simulink library "arducopter_library"  (R2015a)
settings: Solver=ode45  StartTime=0.0  StopTime=10.0  RelTol=1e-3
values from neighbouring files (symbols this model uses):
  dt = 0.01    [arducopter_initialization.m]    (also in startup.m)
  use_ff = true    [arducopter_initialization.m]    (also in startup.m)
undefined symbols (not defined in the file or in its folder): P
libraries: simulink x3, arducopter_library x2
settings Model: CovSaveCumulativeToWorkspaceVar=on  Creator=anne  LastModifiedBy=pa872d
settings DataIOCC: SaveFormat=Dataset
settings HardwareCC: ProdBitPerPointer=64  ProdLargestAtomicFloat=Float  ProdIntDivRoundTo=Zero  ProdEndianess=LittleEndian  ProdHWDeviceType=Specified
settings ModelReferenceCC: PropagateSignalLabelsOutOfModel=on

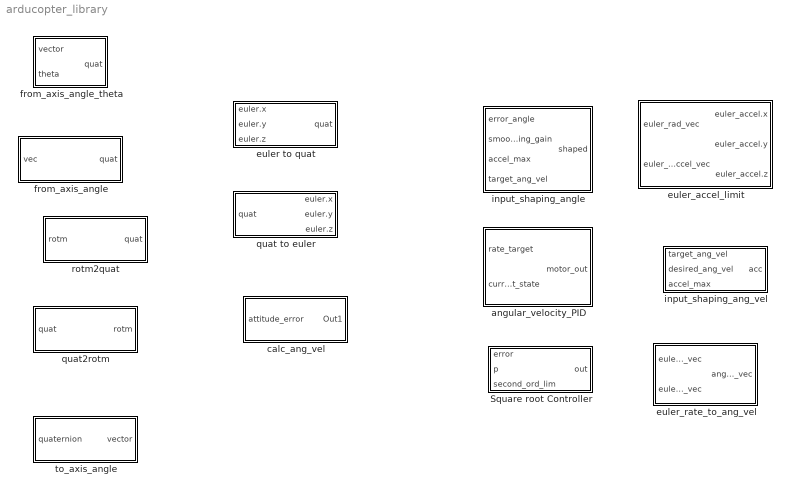
== system arducopter_library ==
  Square root Controller : Subsystem
  angular_velocity_PID : Subsystem  mask(The pid controller for angular velocity){P_rate=0, I_rate=0, D_rate=0, N=0}
      mask prompts: P_rate "P rate"; I_rate "I rate"; D_rate "D rate"; N "Filter Hz"
      mask DialogControl Control3 Prompt: Angular Velocity PID
  calc_ang_vel : Subsystem
  euler to quat : Subsystem
  euler_accel_limit : Subsystem
  euler_rate_to_ang_vel : Subsystem
  from_axis_angle : Subsystem
  from_axis_angle_theta : MATLAB Function  TreatAsAtomicUnit=on
      settings: PermitHierarchicalResolution=ParametersOnly
  input_shaping_ang_vel : Subsystem
  input_shaping_angle : Subsystem
  quat to euler : Subsystem
  quat2rotm : Subsystem
  rotm2quat : Subsystem
  "to_axis_angle " : Subsystem

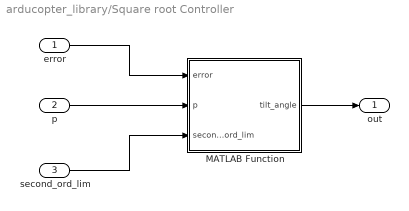
== system arducopter_library/Square root Controller ==
  error : Inport
  p : Inport  Port=2
  second_ord_lim : Inport  Port=3
  MATLAB Function : MATLAB Function  TreatAsAtomicUnit=on
      settings: PermitHierarchicalResolution=ParametersOnly
  out : Outport
  wires:
  error/1 -> MATLAB Function/1(error)
  p/1 -> MATLAB Function/2(p)
  second_ord_lim/1 -> MATLAB Function/3(second_ord_lim)
  MATLAB Function/1(tilt_angle) -> out/1

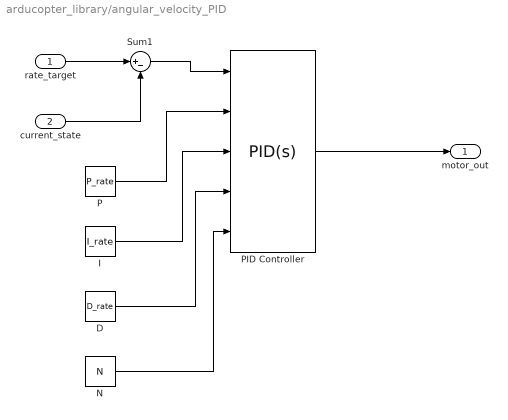
== system arducopter_library/angular_velocity_PID ==
  rate_target : Inport
  current_state : Inport  Port=2
  D : Constant  Value=D_rate
  I : Constant  Value=I_rate
  N : Constant  Value=N
  P : Constant  Value=P_rate
  PID Controller : simulink/Continuous/PID Controller  Controller=PID  TimeDomain=Continuous-time  SampleTime=-1  IntegratorMethod=Forward Euler  FilterMethod=Forward Euler  Form=Parallel  UseFilter=on  ControllerParametersSource=external  P=1  I=1  D=0  N=100  InitialConditionSource=internal  InitialConditionForIntegrator=0  InitialConditionForFilter=0  ExternalReset=none  LimitOutput=off  UpperSaturationLimit=inf  LowerSaturationLimit=-inf  LinearizeAsGain=on  AntiWindupMode=none  Kb=1  TrackingMode=off  Kt=1  PParamMin=[]  PParamMax=[]  IParamMin=[]  IParamMax=[]  DParamMin=[]  DParamMax=[]  NParamMin=[]  NParamMax=[]  KbParamMin=[]  KbParamMax=[]  KtParamMin=[]  KtParamMax=[]  POutMin=[]  POutMax=[]  IOutMin=[]  IOutMax=[]  DOutMin=[]  DOutMax=[]  NOutMin=[]  NOutMax=[]  KbOutMin=[]  KbOutMax=[]  KtOutMin=[]  KtOutMax=[]  IntegratorOutMin=[]  IntegratorOutMax=[]  FilterOutMin=[]  FilterOutMax=[]  SumOutMin=[]  SumOutMax=[]  SumI1OutMin=[]  SumI1OutMax=[]  SumI2OutMin=[]  SumI2OutMax=[]  SumI3OutMin=[]  SumI3OutMax=[]  SumDOutMin=[]  SumDOutMax=[]  SaturationOutMin=[]  SaturationOutMax=[]  IntegratorContinuousStateAttributes=''  IntegratorStateMustResolveToSignalObject=off  IntegratorRTWStateStorageClass=Auto  FilterContinuousStateAttributes=''  FilterStateMustResolveToSignalObject=off  FilterRTWStateStorageClass=Auto  DifferentiatorICPrevScaledInput=0  DifferentiatorOutMin=[]  DifferentiatorOutMax=[]
  Sum1 : Sum  Inputs=|+-
  motor_out : Outport
  wires:
  rate_target/1 -> Sum1/1
  Sum1/1 -> PID Controller/1
  current_state/1 -> Sum1/2
  P/1 -> PID Controller/2
  I/1 -> PID Controller/3
  D/1 -> PID Controller/4
  N/1 -> PID Controller/5
  PID Controller/1 -> motor_out/1

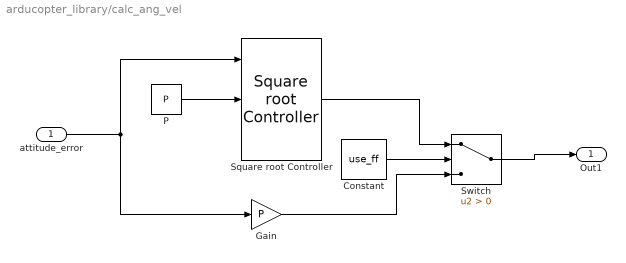
== system arducopter_library/calc_ang_vel ==
  attitude_error : Inport
  Constant : Constant  Value=use_ff
  Gain : Gain  Gain=P
  P : Constant  Value=P
  Square root Controller : arducopter_library/Square root Controller  SystemSampleTime=-1
  Switch : Switch  Criteria=u2 > Threshold
  Out1 : Outport
  wires:
  Square root Controller/1 -> Switch/1
  attitude_error/1 -> Square root Controller/1, Gain/1
  Gain/1 -> Switch/3
  Switch/1 -> Out1/1
  Constant/1 -> Switch/2
  P/1 -> Square root Controller/2

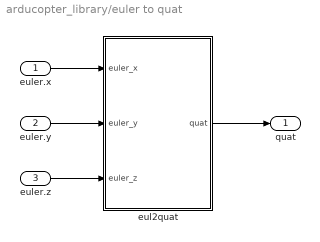
== system arducopter_library/euler to quat ==
  euler.x : Inport
  euler.y : Inport  Port=2
  euler.z : Inport  Port=3
  eul2quat : MATLAB Function  TreatAsAtomicUnit=on
      settings: PermitHierarchicalResolution=ParametersOnly
  quat : Outport
  wires:
  eul2quat/1(quat) -> quat/1
  euler.x/1 -> eul2quat/1(euler_x)
  euler.y/1 -> eul2quat/2(euler_y)
  euler.z/1 -> eul2quat/3(euler_z)

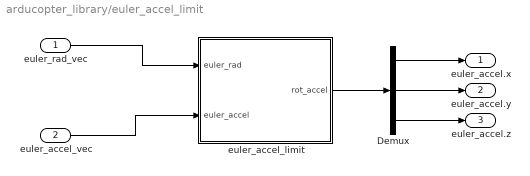
== system arducopter_library/euler_accel_limit ==
  euler_rad_vec : Inport
  euler_accel_vec : Inport  Port=2
  Demux : Demux  Outputs=3
  euler_accel_limit : MATLAB Function  TreatAsAtomicUnit=on
      settings: PermitHierarchicalResolution=ParametersOnly
  euler_accel.x : Outport
  euler_accel.y : Outport  Port=2
  euler_accel.z : Outport  Port=3
  wires:
  euler_accel_limit/1(rot_accel) -> Demux/1
  Demux/1 -> euler_accel.x/1
  Demux/2 -> euler_accel.y/1
  Demux/3 -> euler_accel.z/1
  euler_rad_vec/1 -> euler_accel_limit/1(euler_rad)
  euler_accel_vec/1 -> euler_accel_limit/2(euler_accel)

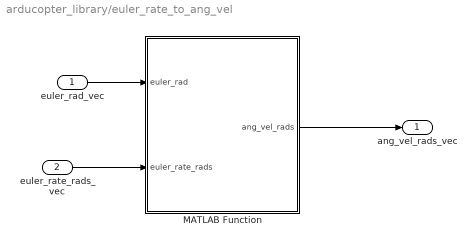
== system arducopter_library/euler_rate_to_ang_vel ==
  euler_rad_vec : Inport
  euler_rate_rads_vec : Inport  Port=2
  MATLAB Function : MATLAB Function  TreatAsAtomicUnit=on
      settings: PermitHierarchicalResolution=ParametersOnly
  ang_vel_rads_vec : Outport
  wires:
  euler_rate_rads_vec/1 -> MATLAB Function/2(euler_rate_rads)
  euler_rad_vec/1 -> MATLAB Function/1(euler_rad)
  MATLAB Function/1(ang_vel_rads) -> ang_vel_rads_vec/1

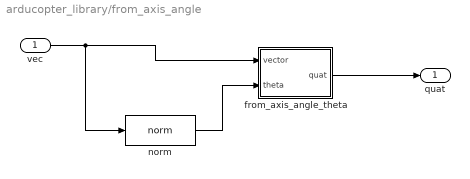
== system arducopter_library/from_axis_angle ==
  vec : Inport
  from_axis_angle_theta : MATLAB Function  TreatAsAtomicUnit=on
      settings: PermitHierarchicalResolution=ParametersOnly
  "norm " : MATLABFcn  MATLABFcn=norm
  quat : Outport
  wires:
  vec/1 -> "norm "/1, from_axis_angle_theta/1(vector)
  "norm "/1 -> from_axis_angle_theta/2(theta)
  from_axis_angle_theta/1(quat) -> quat/1

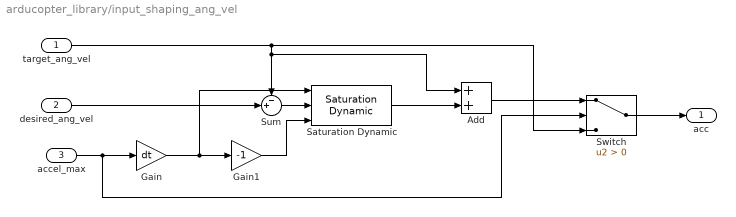
== system arducopter_library/input_shaping_ang_vel ==
  target_ang_vel : Inport
  desired_ang_vel : Inport  Port=2
  accel_max : Inport  Port=3
  Add : Sum
  Gain : Gain  Gain=dt
  Gain1 : Gain  Gain=-1
  Saturation Dynamic : simulink/Discontinuities/Saturation Dynamic  OutMin=[]  OutMax=[]  OutDataTypeStr=Inherit: Same as second input  OutDataType=fixdt(1, 16)  OutScaling=2^-10  DoSatur=off
  Sum : Sum  Inputs=-+|
  Switch : Switch  Criteria=u2 > Threshold
  acc : Outport
  wires:
  accel_max/1 -> Switch/2, Gain/1
  desired_ang_vel/1 -> Sum/2
  target_ang_vel/1 -> Switch/3, Add/1, Sum/1
  Sum/1 -> Saturation Dynamic/2
  Saturation Dynamic/1 -> Add/2
  Gain/1 -> Saturation Dynamic/1, Gain1/1
  Gain1/1 -> Saturation Dynamic/3
  Add/1 -> Switch/1
  Switch/1 -> acc/1

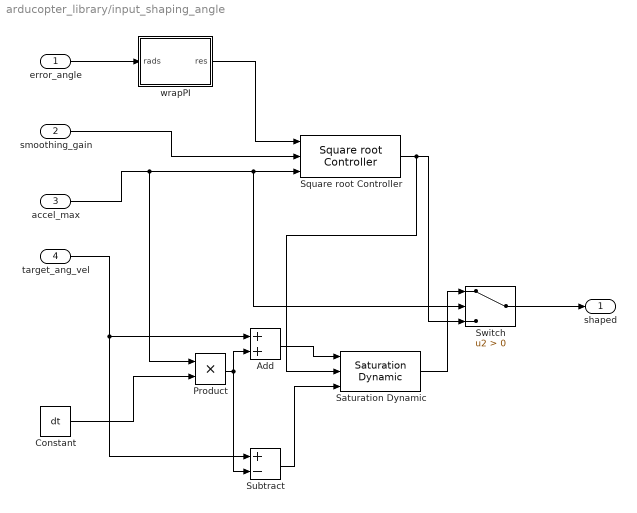
== system arducopter_library/input_shaping_angle ==
  error_angle : Inport
  smoothing_gain : Inport  Port=2
  accel_max : Inport  Port=3
  target_ang_vel : Inport  Port=4
  Add : Sum
  Constant : Constant  Value=dt
  Product : Product
  Saturation Dynamic : simulink/Discontinuities/Saturation Dynamic  OutMin=[]  OutMax=[]  OutDataTypeStr=Inherit: Same as second input  OutDataType=fixdt(1, 16)  OutScaling=2^-10  DoSatur=off
  Square root Controller : arducopter_library/Square root Controller  SystemSampleTime=-1
  Subtract : Sum  Inputs=+-
  Switch : Switch  Criteria=u2 > Threshold
  wrapPI : MATLAB Function  TreatAsAtomicUnit=on
      settings: PermitHierarchicalResolution=ParametersOnly
  shaped : Outport
  wires:
  error_angle/1 -> wrapPI/1(rads)
  wrapPI/1(res) -> Square root Controller/1
  smoothing_gain/1 -> Square root Controller/2
  accel_max/1 -> Switch/2, Square root Controller/3, Product/1
  Square root Controller/1 -> Saturation Dynamic/2, Switch/3
  Constant/1 -> Product/2
  target_ang_vel/1 -> Add/1, Subtract/1
  Product/1 -> Add/2, Subtract/2
  Subtract/1 -> Saturation Dynamic/3
  Add/1 -> Saturation Dynamic/1
  Saturation Dynamic/1 -> Switch/1
  Switch/1 -> shaped/1

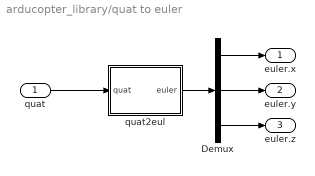
== system arducopter_library/quat to euler ==
  quat : Inport
  Demux : Demux  Outputs=3
  quat2eul : MATLAB Function  TreatAsAtomicUnit=on
      settings: PermitHierarchicalResolution=ParametersOnly
  euler.x : Outport
  euler.y : Outport  Port=2
  euler.z : Outport  Port=3
  wires:
  quat/1 -> quat2eul/1(quat)
  quat2eul/1(euler) -> Demux/1
  Demux/2 -> euler.y/1
  Demux/1 -> euler.x/1
  Demux/3 -> euler.z/1

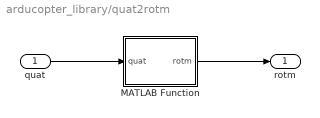
== system arducopter_library/quat2rotm ==
  quat : Inport
  MATLAB Function : MATLAB Function  TreatAsAtomicUnit=on
      settings: PermitHierarchicalResolution=ParametersOnly
  rotm : Outport
  wires:
  quat/1 -> MATLAB Function/1(quat)
  MATLAB Function/1(rotm) -> rotm/1

== system arducopter_library/rotm2quat ==
  rotm : Inport
  MATLAB Function : MATLAB Function  TreatAsAtomicUnit=on
      settings: PermitHierarchicalResolution=ParametersOnly
  quat : Outport
  wires:
  rotm/1 -> MATLAB Function/1(rotm)
  MATLAB Function/1(quat) -> quat/1

== system arducopter_library/to_axis_angle  ==
  quaternion : Inport
  to_axis_angle : MATLAB Function  TreatAsAtomicUnit=on
      settings: PermitHierarchicalResolution=ParametersOnly
  vector : Outport
  wires:
  quaternion/1 -> to_axis_angle/1(quat)
  to_axis_angle/1(vec) -> vector/1

== matlab function arducopter_library/euler to quat/eul2quat ==
  data: euler_x input; quat output; euler_y input; euler_z input
function quat = fcn(euler_x, euler_y, euler_z)
% Eul to quat with zyx order
quat = eul2quat([euler_z, euler_y, euler_x]);

== matlab function arducopter_library/Square root Controller/MATLAB Function ==
  data: error input; tilt_angle output; p input; second_ord_lim input
function tilt_angle = sqr_ctrl(error, p, second_ord_lim)
    if second_ord_lim <= 0 || p==0
        tilt_angle = error * p;
        return
    end
    
    linear_dist = second_ord_lim/(p^2);
    
    if error > linear_dist
        tilt_angle = sqrt(2*second_ord_lim*(error-(linear_dist/2)));
        return
    elseif error < -linear_dist
        tilt_angle = sqrt(2*second_ord_lim*(-error-(linear_dist/2)));
        return
    else
        tilt_angle = error * p;
        return
    end
end

== matlab function arducopter_library/quat to euler/quat2eul ==
  data: quat input; euler output
function euler = fcn(quat)
% Calculate the eulers in ZYX, and flip for [roll, pitch, yaw]
euler = flip(quat2eul(quat));

== matlab function arducopter_library/euler_accel_limit/euler_accel_limit ==
  data: euler_rad input; rot_accel output; euler_accel input
function rot_accel = fcn(euler_rad, euler_accel)
% This represents the AC_AttitudeControl::euler_accel_limit function
% Translates body frame acceleration limits to the euler axis

rot_accel = [euler_accel(1), 0, 0];
if euler_accel(1)<=0 || euler_accel(2)<=0 || euler_accel(3)<=0
    rot_accel(2) = euler_accel(2);
    rot_accel(3) = euler_accel(3);
else
    sin_phi = min(max(abs(sin(euler_rad(1))), 0.1), 1);
    cos_phi = min(max(abs(cos(euler_rad(1))), 0.1), 1);
    sin_theta = min(max(abs(sin(euler_rad(2))), 0.1), 1);
    
    rot_accel(2) = min(euler_accel(2)/cos_phi, euler_accel(3)/sin_phi);
    rot_accel(3) = min(min(euler_accel(1)/sin_theta, euler_accel(2)/sin_phi),...
                    euler_accel(3)/cos_phi);
end

return

== matlab function arducopter_library/input_shaping_angle/wrapPI ==
  data: rads input; res output
function res = fcn(rads)
% wraps radians within -pi and pi
res = mod(rads, 2*pi);

if res > pi
    res = res - 2*pi;
end

return

== matlab function arducopter_library/euler_rate_to_ang_vel/MATLAB Function ==
  data: euler_rad input; ang_vel_rads output; euler_rate_rads input
function ang_vel_rads = euler_rate_to_ang_vel(euler_rad, euler_rate_rads)
% Convert a 321-intristic euler angle derivative to an angular velocity
% vector

sin_theta = sin(euler_rad(2));
cos_theta = cos(euler_rad(2));
sin_phi = sin(euler_rad(1));
cos_phi = cos(euler_rad(1));

ang_vel_rads = [0, 0, 0];

ang_vel_rads(1) = euler_rate_rads(1) - sin_theta * euler_rate_rads(3);
ang_vel_rads(2) = cos_phi * euler_rate_rads(2) + sin_phi * cos_theta * euler_rate_rads(3);
ang_vel_rads(3) = -sin_phi * euler_rate_rads(2) + cos_theta * cos_phi * euler_rate_rads(3);

return

== matlab function arducopter_library/rotm2quat/MATLAB Function ==
  data: rotm input; quat output
function quat = fcn(rotm)
quat = rotm2quat(rotm);

== matlab function arducopter_library/quat2rotm/MATLAB Function ==
  data: quat input; rotm output
function rotm = fcn(quat)
rotm = quat2rotm(quat);

== matlab function arducopter_library/from_axis_angle_theta ==
  data: vector input; quat output; theta input
function quat = fcn(vector, theta)
% create rotation matrix for rotation about the vector v by angle theta
theta = sqrt(vector(1)^2 + vector(2)^2 + vector(3)^2);

if (theta == 0)
    quat = [1 0 0 0];
else
    vector = vector / theta;
    st2 = sin(theta/2);
    quat = [cos(theta/2),
            vector(1) * st2,
            vector(2) * st2,
            vector(3) * st2];
end

== matlab function arducopter_library/from_axis_angle/from_axis_angle_theta ==
  data: vector input; quat output; theta input
function quat = fcn(vector, theta)
% create rotation matrix for rotation about the vector v by angle theta
if (theta == 0)
    quat = [1 0 0 0];
else
    vector = vector / theta;
    st2 = sin(theta/2);
    quat = [cos(theta/2),
            vector(1) * st2,
            vector(2) * st2,
            vector(3) * st2];
end

== matlab function arducopter_library/to_axis_angle /to_axis_angle ==
  data: quat input; vec output
function vec = to_axis_angle(quat)
l = norm([quat(2) quat(3) quat(4)]);
vec = [quat(2) quat(3) quat(4)];
if l
    vec = vec/l;
    res = mod(2*atan2(l, quat(1)), 2*pi);
    if res > pi
        res = res - 2*pi;
    end
    vec = vec * res;
end
return
